simulink model "gm_sampleModel1972_3_sub"  (R2023a)
settings: Solver=VariableStepAuto  StartTime=0.0  StopTime=10.0  RelTol=1e-3
settings Model: Creator=user1  LastModifiedBy=user1
settings OptimizationCC: BlockReduction=off  ConditionallyExecuteInputs=off
settings DebuggingCC: InheritedTsInSrcMsg=none

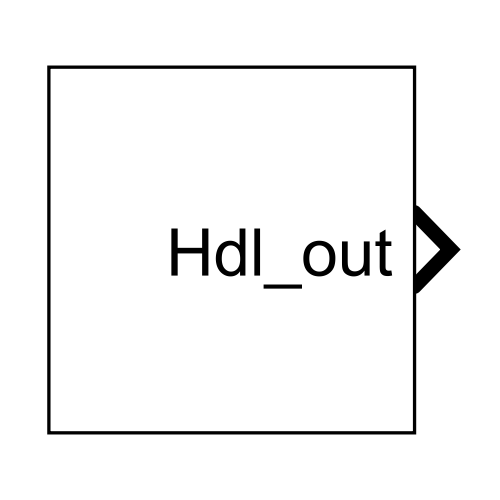
[thumbnail: Simulink's stored preview of the top-level diagram]
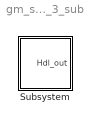
== system gm_sampleModel1972_3_sub ==
  Subsystem : Subsystem

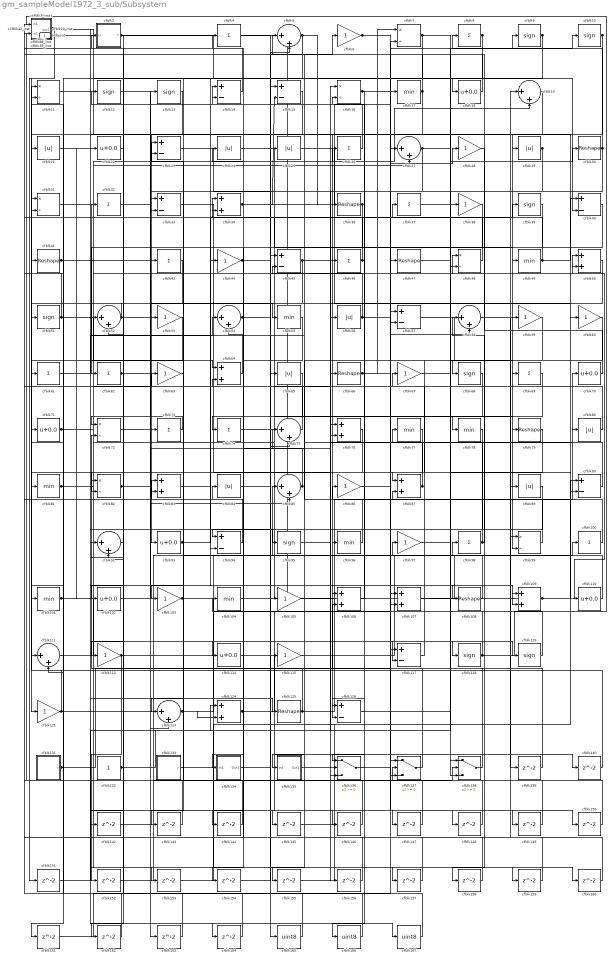
== system gm_sampleModel1972_3_sub/Subsystem ==
  cfblk1 : Constant  Value=0  OutDataTypeStr=uint8  SampleTime=1
  cfblk{9..10,12..13,39,51,68,95,118..119} (10 alike) : Signum
  cfblk{4,8,26,32,37,43,46,61..62,69,73..74,98,100} (14 alike) : Sum  Inputs=+  OutDataTypeStr=uint8
  cfblk{17,49,55,77..78,81,96,101,104} (9 alike) : MinMax  OutDataTypeStr=uint8
  cfblk{18,22,70..71,93,102,110,114} (8 alike) : Bias  Bias=0.0  SaturateOnIntegerOverflow=off
  cfblk{6,28,38,44,53,59..60,63,67,86,97,103,105,112,115,121} (16 alike) : Gain  OutDataTypeStr=uint8
  cfblk{34,50,64,76,83,87,106..107,109,124} (10 alike) : Sum  OutDataTypeStr=uint8
  cfblk{30,36,41,47,66,79,108,125} (8 alike) : Reshape
  cfblk{7,11,16,31,48,72,82,99} (8 alike) : Product  Inputs=*/  OutDataTypeStr=uint8  RndMeth=Zero  SaturateOnIntegerOverflow=on
  cfblk{5,19,27,52,54,58,75,85,92,111,123} (11 alike) : Sum  Inputs=|++  OutDataTypeStr=uint8
  cfblk113_inst : Subsystem
  cfblk116_inst : Subsystem
  cfblk{14..15,23,33,40,45,57,90,94,117,126} (11 alike) : Sum  Inputs=+-  OutDataTypeStr=uint8
  cfblk120_inst : Subsystem
  cfblk122_inst : Subsystem
  cfblk131 : Subsystem  mask(Counter Limited){uplimit=double(7), tsamp=double(-1)}
      mask prompts: uplimit "Simulink:masks:UpperLimit_MP"; tsamp "Simulink:masks:SampleTime_MP"
      mask help: Simulink:masks:CounterLimited_MD
      mask init:
      | nbits = double(8);
      | tsamp = double(-1);
      | uplimit = double(7);
  cfblk132 : Constant  OutDataTypeStr=uint8  SampleTime=-1
  cfblk133 : Subsystem  mask(Counter Free-Running){NumBits=double(16), tsamp=double(-1)}
      mask prompts: NumBits "Simulink:masks:NumberOfBits_MP"; tsamp "Simulink:masks:SampleTime_MP"
      mask help: Simulink:masks:CounterFreeRunning_MD
  cfblk134 : Subsystem
  cfblk135 : Subsystem
  cfblk136 : Switch  OutDataTypeStr=uint8  SaturateOnIntegerOverflow=off  InputSameDT=off
  cfblk137 : Switch  OutDataTypeStr=uint8  SaturateOnIntegerOverflow=off  InputSameDT=off
  cfblk138 : Switch  OutDataTypeStr=uint8  SaturateOnIntegerOverflow=off  InputSameDT=off
  cfblk{139..140,142..164} (25 alike) : Delay  SampleTime=1
  cfblk165 : DataTypeConversion  OutDataTypeStr=uint8  SaturateOnIntegerOverflow=off  RndMeth=Floor
  cfblk166 : DataTypeConversion  OutDataTypeStr=uint8  SaturateOnIntegerOverflow=off  RndMeth=Floor
  cfblk167 : DataTypeConversion  OutDataTypeStr=uint8  SaturateOnIntegerOverflow=off  RndMeth=Floor
  cfblk2 : Subsystem  mask(Detect Fall Negative){vinit=double(0), InputProcessing=Elements as channels (sample based), OutDataTypeStr=uint8}
      mask prompts: vinit "Simulink:masks:InitialCondition_MP"; InputProcessing "Simulink:masks:InputProcessing_MP"; OutDataTypeStr "Simulink:masks:OutputDataType_MP"
      mask help: Simulink:masks:DetectFallNegative_MD
      mask init:
      | InputProcessing = 'Elements as channels (sample based)';
      | OutDataTypeStr = 'uint8';
      | vinit = double(0);
      mask TypeOptions InputProcessing: Simulink:masks:ColumnsAsChannelsFrameBased | Simulink:masks:ElementsAsChannelsSampleBased
      mask TypeOptions OutDataTypeStr: Simulink:masks:uint8 | Simulink:masks:boolean
      mask Display: fprintf('U < 0\n&  NOT\nU/z < 0')
  cfblk20_inst : Subsystem
  cfblk{21,24..25,29,56,65,80,84,89} (9 alike) : Abs  OutDataTypeStr=uint8  SaturateOnIntegerOverflow=off
  cfblk35_inst : Subsystem
  cfblk3_inst : Subsystem
  cfblk42_inst : Subsystem
  cfblk88_inst : Subsystem
  Hdl_out : Outport  OutDataTypeStr=uint8  SampleTime=1
  wires:
  cfblk1/1 -> cfblk121/1
  cfblk10/1 -> cfblk93/1, cfblk126/2
  cfblk100/1 -> cfblk86/1
  cfblk101/1 -> cfblk22/1, cfblk19/2, cfblk160/1
  cfblk102/1 -> cfblk13/1
  cfblk103/1 -> cfblk117/2, cfblk157/1
  cfblk104/1 -> cfblk37/1
  cfblk105/1 -> cfblk70/1
  cfblk106/1 -> cfblk16/2
  cfblk107/1 -> cfblk100/1
  cfblk108/1 -> cfblk85/1
  cfblk109/1 -> cfblk50/1, Hdl_out/1
  cfblk11/1 -> cfblk99/2
  cfblk110/1 -> cfblk63/1
  cfblk111/1 -> cfblk48/1
  cfblk112/1 -> cfblk97/1, cfblk152/1
  cfblk113_inst/1(out1) -> cfblk123/2, cfblk105/1
  cfblk114/1 -> cfblk140/1
  cfblk115/1 -> cfblk98/1
  cfblk116_inst/1(out1) -> cfblk60/1
  cfblk117/1 -> cfblk67/1
  cfblk118/1 -> cfblk113_inst/1(in1), cfblk104/1
  cfblk119/1 -> cfblk84/1
  cfblk12/1 -> cfblk73/1
  cfblk120_inst/1(out1) -> cfblk137/1
  cfblk121/1 -> cfblk76/2, cfblk19/1, cfblk11/1
  cfblk122_inst/1(out1) -> cfblk165/1
  cfblk123/1 -> cfblk57/2, cfblk124/2
  cfblk124/1 -> cfblk66/1, cfblk147/1
  cfblk125/1 -> cfblk87/2, cfblk12/1
  cfblk126/1 -> cfblk38/1
  cfblk13/1 -> cfblk21/1
  cfblk131/1(y) -> cfblk71/1, cfblk57/1
  cfblk132/1 -> cfblk56/1, cfblk48/2
  cfblk133/1(y) -> cfblk59/1
  cfblk134/1(Out1) -> cfblk75/2
  cfblk135/1(Out1) -> cfblk17/1
  cfblk136/1 -> cfblk28/1
  cfblk137/1 -> cfblk72/2
  cfblk138/1 -> cfblk14/1
  cfblk139/1 -> cfblk106/2
  cfblk14/1 -> cfblk35_inst/1(in1)
  cfblk140/1 -> cfblk111/1
  cfblk142/1 -> cfblk16/1
  cfblk143/1 -> cfblk20_inst/1(in1)
  cfblk144/1 -> cfblk83/1
  cfblk145/1 -> cfblk90/1
  cfblk146/1 -> cfblk120_inst/2(in2)
  cfblk147/1 -> cfblk117/1
  cfblk148/1 -> cfblk113_inst/2(in2)
  cfblk149/1 -> cfblk23/1
  cfblk15/1 -> cfblk111/2
  cfblk150/1 -> cfblk14/2
  cfblk151/1 -> cfblk124/1
  cfblk152/1 -> cfblk138/2
  cfblk153/1 -> cfblk5/2
  cfblk154/1 -> cfblk15/1
  cfblk155/1 -> cfblk137/2
  cfblk156/1 -> cfblk116_inst/2(in2)
  cfblk157/1 -> cfblk52/2
  cfblk158/1 -> cfblk34/1
  cfblk159/1 -> cfblk99/1
  cfblk16/1 -> cfblk136/1, cfblk49/1
  cfblk160/1 -> cfblk3_inst/2(in2)
  cfblk161/1 -> cfblk27/1
  cfblk162/1 -> cfblk31/1
  cfblk163/1 -> cfblk88_inst/2(in2)
  cfblk164/1 -> cfblk11/2
  cfblk165/1 -> cfblk92/1
  cfblk166/1 -> cfblk122_inst/1(in1)
  cfblk167/1 -> cfblk122_inst/2(in2)
  cfblk17/1 -> cfblk5/1, cfblk82/2
  cfblk18/1 -> cfblk42_inst/2(in2)
  cfblk19/1 -> cfblk53/1
  cfblk2/1(Y) -> cfblk40/2, cfblk142/1
  cfblk20_inst/1(out1) -> cfblk45/1
  cfblk21/1 -> cfblk109/2
  cfblk22/1 -> cfblk102/1
  cfblk23/1 -> cfblk115/1
  cfblk24/1 -> cfblk107/1
  cfblk25/1 -> cfblk110/1
  cfblk26/1 -> cfblk2/1(U)
  cfblk27/1 -> cfblk90/2, cfblk136/3
  cfblk28/1 -> cfblk158/1
  cfblk29/1 -> cfblk68/1, cfblk78/1
  cfblk3_inst/1(out1) -> cfblk23/2, cfblk164/1
  cfblk30/1 -> cfblk33/2, cfblk8/1
  cfblk31/1 -> cfblk27/2
  cfblk32/1 -> cfblk167/1
  cfblk33/1 -> cfblk156/1
  cfblk34/1 -> cfblk15/2, cfblk7/2
  cfblk35_inst/1(out1) -> cfblk64/1, cfblk153/1
  cfblk36/1 -> cfblk136/2, cfblk43/1
  cfblk37/1 -> cfblk10/1
  cfblk38/1 -> cfblk54/2
  cfblk39/1 -> cfblk162/1
  cfblk4/1 -> cfblk25/1
  cfblk40/1 -> cfblk62/1
  cfblk41/1 -> cfblk145/1, cfblk55/1
  cfblk42_inst/1(out1) -> cfblk151/1, cfblk150/1, cfblk149/1
  cfblk43/1 -> cfblk83/2
  cfblk44/1 -> cfblk65/1, cfblk74/1
  cfblk45/1 -> cfblk138/1, cfblk81/1
  cfblk46/1 -> cfblk24/1, cfblk96/1
  cfblk47/1 -> cfblk69/1
  cfblk48/1 -> cfblk88_inst/1(in1)
  cfblk49/1 -> cfblk40/1, cfblk3_inst/1(in1)
  cfblk5/1 -> cfblk92/2, cfblk36/1
  cfblk50/1 -> cfblk143/1
  cfblk51/1 -> cfblk20_inst/2(in2), cfblk163/1
  cfblk52/1 -> cfblk85/2, cfblk51/1
  cfblk53/1 -> cfblk161/1
  cfblk54/1 -> cfblk146/1, cfblk26/1
  cfblk55/1 -> cfblk144/1
  cfblk56/1 -> cfblk58/2, cfblk45/2
  cfblk57/1 -> cfblk89/1
  cfblk58/1 -> cfblk139/1
  cfblk59/1 -> cfblk87/1
  cfblk6/1 -> cfblk47/1, cfblk148/1
  cfblk60/1 -> cfblk135/1(In1)
  cfblk61/1 -> cfblk54/1
  cfblk62/1 -> cfblk50/2, cfblk107/2
  cfblk63/1 -> cfblk103/1
  cfblk64/1 -> cfblk32/1
  cfblk65/1 -> cfblk134/1(In1)
  cfblk66/1 -> cfblk9/1, cfblk7/1
  cfblk67/1 -> cfblk30/1
  cfblk68/1 -> cfblk155/1
  cfblk69/1 -> cfblk94/1
  cfblk7/1 -> cfblk94/2, cfblk29/1
  cfblk70/1 -> cfblk116_inst/1(in1)
  cfblk71/1 -> cfblk95/1, cfblk33/1
  cfblk72/1 -> cfblk118/1
  cfblk73/1 -> cfblk72/1
  cfblk74/1 -> cfblk79/1
  cfblk75/1 -> cfblk35_inst/2(in2)
  cfblk76/1 -> cfblk101/1
  cfblk77/1 -> cfblk166/1
  cfblk78/1 -> cfblk154/1
  cfblk79/1 -> cfblk137/3
  cfblk8/1 -> cfblk18/1, cfblk123/1
  cfblk80/1 -> cfblk41/1
  cfblk81/1 -> cfblk125/1, cfblk114/1, cfblk44/1, cfblk46/1
  cfblk82/1 -> cfblk76/1, cfblk159/1
  cfblk83/1 -> cfblk108/1
  cfblk84/1 -> cfblk6/1
  cfblk85/1 -> cfblk64/2, cfblk4/1
  cfblk86/1 -> cfblk80/1
  cfblk87/1 -> cfblk82/1, cfblk31/2
  cfblk88_inst/1(out1) -> cfblk106/1
  cfblk89/1 -> cfblk126/1
  cfblk9/1 -> cfblk138/3, cfblk61/1
  cfblk90/1 -> cfblk120_inst/1(in1)
  cfblk92/1 -> cfblk112/1
  cfblk93/1 -> cfblk39/1, cfblk109/1
  cfblk94/1 -> cfblk42_inst/1(in1)
  cfblk95/1 -> cfblk77/1
  cfblk96/1 -> cfblk75/1
  cfblk97/1 -> cfblk119/1
  cfblk98/1 -> cfblk58/1, cfblk52/1
  cfblk99/1 -> cfblk34/2

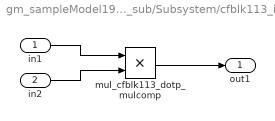
== system gm_sampleModel1972_3_sub/Subsystem/cfblk113_inst ==
  in1 : Inport  OutDataTypeStr=uint8  SampleTime=1
  in2 : Inport  Port=2  OutDataTypeStr=uint8  SampleTime=1
  mul_cfblk113_dotp_mulcomp : Product  Inputs=**  OutDataTypeStr=uint8  SampleTime=1
  out1 : Outport  OutDataTypeStr=uint8  SampleTime=1
  wires:
  in1/1 -> mul_cfblk113_dotp_mulcomp/1
  in2/1 -> mul_cfblk113_dotp_mulcomp/2
  mul_cfblk113_dotp_mulcomp/1 -> out1/1

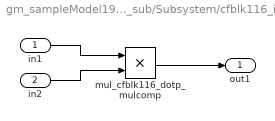
== system gm_sampleModel1972_3_sub/Subsystem/cfblk116_inst ==
  in1 : Inport  OutDataTypeStr=uint8  SampleTime=1
  in2 : Inport  Port=2  OutDataTypeStr=uint8  SampleTime=1
  mul_cfblk116_dotp_mulcomp : Product  Inputs=**  OutDataTypeStr=uint8  SampleTime=1
  out1 : Outport  OutDataTypeStr=uint8  SampleTime=1
  wires:
  in1/1 -> mul_cfblk116_dotp_mulcomp/1
  in2/1 -> mul_cfblk116_dotp_mulcomp/2
  mul_cfblk116_dotp_mulcomp/1 -> out1/1

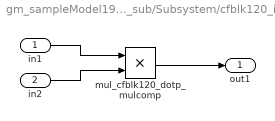
== system gm_sampleModel1972_3_sub/Subsystem/cfblk120_inst ==
  in1 : Inport  OutDataTypeStr=uint8  SampleTime=1
  in2 : Inport  Port=2  OutDataTypeStr=uint8  SampleTime=1
  mul_cfblk120_dotp_mulcomp : Product  Inputs=**  OutDataTypeStr=uint8  SampleTime=1
  out1 : Outport  OutDataTypeStr=uint8  SampleTime=1
  wires:
  in1/1 -> mul_cfblk120_dotp_mulcomp/1
  in2/1 -> mul_cfblk120_dotp_mulcomp/2
  mul_cfblk120_dotp_mulcomp/1 -> out1/1

== system gm_sampleModel1972_3_sub/Subsystem/cfblk122_inst ==
  in1 : Inport  OutDataTypeStr=uint8  SampleTime=1
  in2 : Inport  Port=2  OutDataTypeStr=uint8  SampleTime=1
  mul_cfblk122_dotp_mulcomp : Product  Inputs=**  OutDataTypeStr=uint8  SampleTime=1
  out1 : Outport  OutDataTypeStr=uint8  SampleTime=1
  wires:
  in1/1 -> mul_cfblk122_dotp_mulcomp/1
  in2/1 -> mul_cfblk122_dotp_mulcomp/2
  mul_cfblk122_dotp_mulcomp/1 -> out1/1

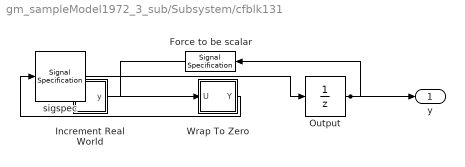
== system gm_sampleModel1972_3_sub/Subsystem/cfblk131 ==
  Force to be scalar : SignalSpecification  DisableCoverage=on  Dimensions=1
  Increment Real World : Subsystem  mask(Real World Value Increment){}
      mask help: Simulink:masks:RealWorldValueIncrement_MD
      mask Display: disp('V++')
  Output : UnitDelay  InitialCondition=0.0  SampleTime=tsamp  HasFrameUpgradeWarning=on
  Wrap To Zero : Subsystem  mask(Wrap To Zero){Threshold=double(7)}
      mask prompts: Threshold "Simulink:masks:Threshold_MP"
      mask help: Simulink:masks:WrapToZero_MD
  sigspec : SignalSpecification  OutDataTypeStr=uint8  Dimensions=1
  y : Outport  SampleTime=1
  wires:
  Force to be scalar/1 -> Increment Real World/1(u)
  Increment Real World/1(y) -> Wrap To Zero/1(U)
  Output/1 -> Force to be scalar/1, y/1
  Wrap To Zero/1(Y) -> sigspec/1
  sigspec/1 -> Output/1

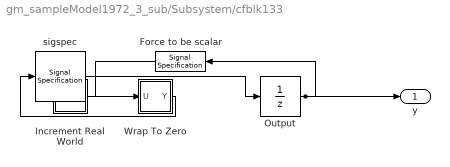
== system gm_sampleModel1972_3_sub/Subsystem/cfblk133 ==
  Force to be scalar : SignalSpecification  DisableCoverage=on  Dimensions=1
  Increment Real World : Subsystem  mask(Real World Value Increment){}
      mask help: Simulink:masks:RealWorldValueIncrement_MD
      mask Display: disp('V++')
  Output : UnitDelay  InitialCondition=0.0  SampleTime=tsamp  HasFrameUpgradeWarning=on
  Wrap To Zero : Subsystem  mask(Wrap To Zero){Threshold=double(65535)}
      mask prompts: Threshold "Simulink:masks:Threshold_MP"
      mask help: Simulink:masks:WrapToZero_MD
  sigspec : SignalSpecification  OutDataTypeStr=uint16  Dimensions=1
  y : Outport  SampleTime=1
  wires:
  Force to be scalar/1 -> Increment Real World/1(u)
  Increment Real World/1(y) -> Wrap To Zero/1(U)
  Output/1 -> Force to be scalar/1, y/1
  Wrap To Zero/1(Y) -> sigspec/1
  sigspec/1 -> Output/1

== system gm_sampleModel1972_3_sub/Subsystem/cfblk134 ==
  In1 : Inport  OutDataTypeStr=uint8  PortDimensions=1  SampleTime=1
  Out1 : Outport  SampleTime=1
  wires:
  In1/1 -> Out1/1

== system gm_sampleModel1972_3_sub/Subsystem/cfblk135 ==
  In1 : Inport  OutDataTypeStr=uint8  PortDimensions=1  SampleTime=1
  Out1 : Outport  SampleTime=1
  wires:
  In1/1 -> Out1/1

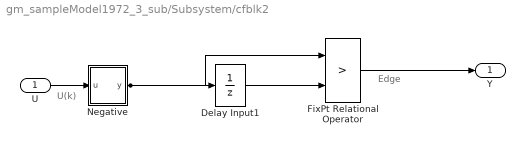
== system gm_sampleModel1972_3_sub/Subsystem/cfblk2 ==
  note: U(k)
  note: Edge
  U : Inport  OutDataTypeStr=uint8  SampleTime=1
  Delay Input1 : UnitDelay  Description=Store in Global RAM  DisableCoverage=on  InitialCondition=vinit  SampleTime=-1  HasFrameUpgradeWarning=on
  FixPt Relational Operator : RelationalOperator  Operator=>  OutDataTypeStr=fixdt(0, 8)  ZeroCross=off  InputSameDT=off
  Negative : Subsystem  mask(Compare To Zero){relop=<, OutDataTypeStr=boolean, ZeroCross=off}
      mask prompts: relop "Simulink:masks:Operator_MP"; OutDataTypeStr "Simulink:masks:OutputDataType_MP"; ZeroCross "Simulink:masks:EnableZerocrossingDetection_MP"
      mask help: Simulink:masks:CompareToZero_MD
      mask init:
      | OutDataTypeStr = 'boolean';
      | ZeroCross = 'off';
      | blkName = 'sampleModel1972_3_sub/Subsystem/cfblk2/Negative';
      | relop = '<';
      | setValue = 'boolean';
      mask TypeOptions relop: == | ~= | < | <= | >= | >
      mask TypeOptions OutDataTypeStr: Simulink:masks:uint8 | Simulink:masks:boolean
      mask Callback ZeroCross: sl('zeroCrossEnable', gcbh);
      mask Display: disp([relop,' 0'])
  Y : Outport  SampleTime=1
  wires:
  U/1 -> Negative/1(u)
  Delay Input1/1 -> FixPt Relational Operator/2
  FixPt Relational Operator/1 -> Y/1
  Negative/1(y) -> FixPt Relational Operator/1, Delay Input1/1

== system gm_sampleModel1972_3_sub/Subsystem/cfblk20_inst ==
  in1 : Inport  OutDataTypeStr=uint8  SampleTime=1
  in2 : Inport  Port=2  OutDataTypeStr=uint8  SampleTime=1
  mul_cfblk20_dotp_mulcomp : Product  Inputs=**  OutDataTypeStr=uint8  SampleTime=1
  out1 : Outport  OutDataTypeStr=uint8  SampleTime=1
  wires:
  in1/1 -> mul_cfblk20_dotp_mulcomp/1
  in2/1 -> mul_cfblk20_dotp_mulcomp/2
  mul_cfblk20_dotp_mulcomp/1 -> out1/1

== system gm_sampleModel1972_3_sub/Subsystem/cfblk35_inst ==
  in1 : Inport  OutDataTypeStr=uint8  SampleTime=1
  in2 : Inport  Port=2  OutDataTypeStr=uint8  SampleTime=1
  mul_cfblk35_dotp_mulcomp : Product  Inputs=**  OutDataTypeStr=uint8  SampleTime=1
  out1 : Outport  OutDataTypeStr=uint8  SampleTime=1
  wires:
  in1/1 -> mul_cfblk35_dotp_mulcomp/1
  in2/1 -> mul_cfblk35_dotp_mulcomp/2
  mul_cfblk35_dotp_mulcomp/1 -> out1/1

== system gm_sampleModel1972_3_sub/Subsystem/cfblk3_inst ==
  in1 : Inport  OutDataTypeStr=uint8  SampleTime=1
  in2 : Inport  Port=2  OutDataTypeStr=uint8  SampleTime=1
  mul_cfblk3_dotp_mulcomp : Product  Inputs=**  OutDataTypeStr=uint8  SampleTime=1
  out1 : Outport  OutDataTypeStr=uint8  SampleTime=1
  wires:
  in1/1 -> mul_cfblk3_dotp_mulcomp/1
  in2/1 -> mul_cfblk3_dotp_mulcomp/2
  mul_cfblk3_dotp_mulcomp/1 -> out1/1

== system gm_sampleModel1972_3_sub/Subsystem/cfblk42_inst ==
  in1 : Inport  OutDataTypeStr=uint8  SampleTime=1
  in2 : Inport  Port=2  OutDataTypeStr=uint8  SampleTime=1
  mul_cfblk42_dotp_mulcomp : Product  Inputs=**  OutDataTypeStr=uint8  SampleTime=1
  out1 : Outport  OutDataTypeStr=uint8  SampleTime=1
  wires:
  in1/1 -> mul_cfblk42_dotp_mulcomp/1
  in2/1 -> mul_cfblk42_dotp_mulcomp/2
  mul_cfblk42_dotp_mulcomp/1 -> out1/1

== system gm_sampleModel1972_3_sub/Subsystem/cfblk88_inst ==
  in1 : Inport  OutDataTypeStr=uint8  SampleTime=1
  in2 : Inport  Port=2  OutDataTypeStr=uint8  SampleTime=1
  mul_cfblk88_dotp_mulcomp : Product  Inputs=**  OutDataTypeStr=uint8  SampleTime=1
  out1 : Outport  OutDataTypeStr=uint8  SampleTime=1
  wires:
  in1/1 -> mul_cfblk88_dotp_mulcomp/1
  in2/1 -> mul_cfblk88_dotp_mulcomp/2
  mul_cfblk88_dotp_mulcomp/1 -> out1/1

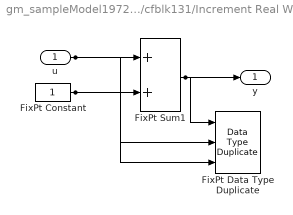
== system gm_sampleModel1972_3_sub/Subsystem/cfblk131/Increment Real World ==
  u : Inport  OutDataTypeStr=uint8  SampleTime=1
  FixPt Constant : Constant  DisableCoverage=on  OutDataTypeStr=Inherit: Inherit via back propagation  SampleTime=-1
  FixPt Data Type Duplicate : DataTypeDuplicate  DisableCoverage=on  NumInputPorts=3
  FixPt Sum1 : Sum  InputSameDT=on  OutDataTypeStr=Inherit: Inherit via back propagation  LockScale=on
  y : Outport  SampleTime=1
  wires:
  u/1 -> FixPt Sum1/1, FixPt Data Type Duplicate/2
  FixPt Constant/1 -> FixPt Sum1/2, FixPt Data Type Duplicate/3
  FixPt Sum1/1 -> FixPt Data Type Duplicate/1, y/1

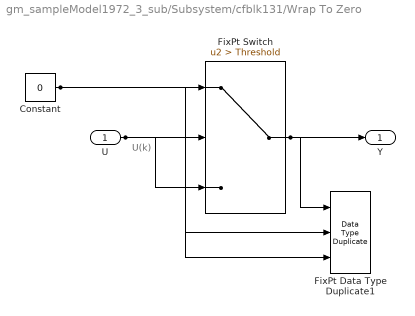
== system gm_sampleModel1972_3_sub/Subsystem/cfblk131/Wrap To Zero ==
  note: U(k)
  U : Inport  OutDataTypeStr=uint8  SampleTime=1
  Constant : Constant  DisableCoverage=on  Value=0  OutDataTypeStr=Inherit: Inherit via back propagation  SampleTime=-1
  FixPt Data Type Duplicate1 : DataTypeDuplicate  DisableCoverage=on  NumInputPorts=3
  FixPt Switch : Switch  Criteria=u2 > Threshold  Threshold=Threshold  OutDataTypeStr=Inherit: Inherit via back propagation  ZeroCross=off  SaturateOnIntegerOverflow=off  InputSameDT=off
  Y : Outport  SampleTime=1
  wires:
  U/1 -> FixPt Switch/3, FixPt Switch/2, FixPt Data Type Duplicate1/2
  Constant/1 -> FixPt Switch/1, FixPt Data Type Duplicate1/3
  FixPt Switch/1 -> FixPt Data Type Duplicate1/1, Y/1

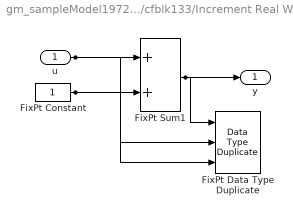
== system gm_sampleModel1972_3_sub/Subsystem/cfblk133/Increment Real World ==
  u : Inport  OutDataTypeStr=uint16  SampleTime=1
  FixPt Constant : Constant  DisableCoverage=on  OutDataTypeStr=Inherit: Inherit via back propagation  SampleTime=-1
  FixPt Data Type Duplicate : DataTypeDuplicate  DisableCoverage=on  NumInputPorts=3
  FixPt Sum1 : Sum  InputSameDT=on  OutDataTypeStr=Inherit: Inherit via back propagation  LockScale=on
  y : Outport  SampleTime=1
  wires:
  u/1 -> FixPt Sum1/1, FixPt Data Type Duplicate/2
  FixPt Constant/1 -> FixPt Sum1/2, FixPt Data Type Duplicate/3
  FixPt Sum1/1 -> FixPt Data Type Duplicate/1, y/1

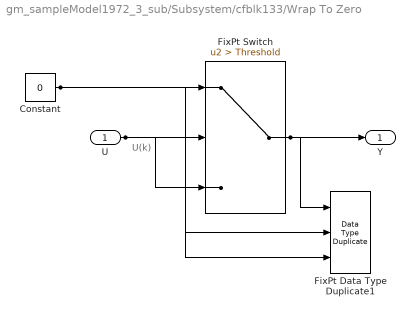
== system gm_sampleModel1972_3_sub/Subsystem/cfblk133/Wrap To Zero ==
  note: U(k)
  U : Inport  OutDataTypeStr=uint16  SampleTime=1
  Constant : Constant  DisableCoverage=on  Value=0  OutDataTypeStr=Inherit: Inherit via back propagation  SampleTime=-1
  FixPt Data Type Duplicate1 : DataTypeDuplicate  DisableCoverage=on  NumInputPorts=3
  FixPt Switch : Switch  Criteria=u2 > Threshold  Threshold=Threshold  OutDataTypeStr=Inherit: Inherit via back propagation  ZeroCross=off  SaturateOnIntegerOverflow=off  InputSameDT=off
  Y : Outport  SampleTime=1
  wires:
  U/1 -> FixPt Switch/3, FixPt Switch/2, FixPt Data Type Duplicate1/2
  Constant/1 -> FixPt Switch/1, FixPt Data Type Duplicate1/3
  FixPt Switch/1 -> FixPt Data Type Duplicate1/1, Y/1

== system gm_sampleModel1972_3_sub/Subsystem/cfblk2/Negative ==
  u : Inport  OutDataTypeStr=uint8  SampleTime=1
  Compare : RelationalOperator  Operator=<  OutDataTypeStr=boolean  ZeroCross=off
  Constant : Constant  DisableCoverage=on  Value=0  OutDataTypeStr=Inherit: Inherit via back propagation  SampleTime=-1  PreserveConstantTs=on
  y : Outport  SampleTime=1
  wires:
  u/1 -> Compare/1
  Compare/1 -> y/1
  Constant/1 -> Compare/2
